simulink model "soccerbot"  (R2017b)
settings: Solver=FixedStepDiscrete  StartTime=0.0  StopTime=10  FixedStep=0.01  RelTol=1e-3
PreLoadFcn:
  | clear;
  | 
  | % Sample times
  | sampleTime = 0.2;
  | 
  | % Control parameters
  | ctrlParam1 = 2;
  | ctrlParam2 = 3.5;
  | 
  | loadIpAddresses;
InitFcn:
  | loadFixedTrajectories;
model workspace (MAT data in the model file):
  SL_ROS_VariableLengthArrays_MaxSizes.CommonInfo.ArrayTruncateAction = 'EmitWarning'
  SL_ROS_VariableLengthArrays_MaxSizes.MsgTypeMap = containers.Map
  SL_ROS_VariableLengthArrays_MaxSizes.MsgTypeMap.serialization.keys = {'sensor_msgs/Image'}
  SL_ROS_VariableLengthArrays_MaxSizes.MsgTypeMap.serialization.values{1}(1).PropertyName = 'Data'
  SL_ROS_VariableLengthArrays_MaxSizes.MsgTypeMap.serialization.values{1}(1).DataType = 'uint8'
  SL_ROS_VariableLengthArrays_MaxSizes.MsgTypeMap.serialization.values{1}(1).MaxLength = 230400
  SL_ROS_VariableLengthArrays_MaxSizes.MsgTypeMap.serialization.values{1}(2).PropertyName = 'Encoding'
  SL_ROS_VariableLengthArrays_MaxSizes.MsgTypeMap.serialization.values{1}(2).DataType = 'uint8'
  SL_ROS_VariableLengthArrays_MaxSizes.MsgTypeMap.serialization.values{1}(2).MaxLength = 128
  SL_ROS_VariableLengthArrays_MaxSizes.MsgTypeMap.serialization.uniformity = 0
  SL_ROS_VariableLengthArrays_MaxSizes.MsgTypeMap.serialization.keyType = 'char'
  SL_ROS_VariableLengthArrays_MaxSizes.MsgTypeMap.serialization.valueType = 'any'
  ctrlParam1 = 1
  ctrlParam2 = 1.5
  sampleTime = 0.01
values from neighbouring files (symbols this model uses):
  findBallTraj = zeros(1000,20)    [loadFixedTrajectories.m]
  getUpBackTraj = getUpBackTraj'    [loadFixedTrajectories.m]
  getUpFrontTraj = getUpFrontTraj'    [loadFixedTrajectories.m]    (also in loadModelData.m)
  motorCalibration = [0;0;0;0;0;0;0;0;0;0;0;0;0;0;0;0;0;0;0;0]    [loadFixedTrajectories.m]    (also in loadRobot.m; soccer_strategy_setup.m)
  prepareToWalkTraj = spline(t, prepareToWalkWayPoints, prepareToWalkTrajTime)'    [loadFixedTrajectories.m]
undefined symbols (not defined in the file or in its folder): customState, DiscIntNeverNeededParam, resting, walkTraj
libraries: simulink x102, robotlib x5, sharedtransform x1, visionsinks x1
(part 1 of 2)
settings Model: Creator=scastro  LastModifiedBy=vuwij
settings OptimizationCC: PassReuseOutputArgsAs=Individual arguments  EfficientMapNaN2IntZero=off  MaxStackSize=64
settings DebuggingCC: ParameterTunabilityLossMsg=error
settings HardwareCC: ProdBitPerPointer=32  ProdBitPerSizeT=32  ProdBitPerPtrDiffT=32  ProdLargestAtomicFloat=None  ProdIntDivRoundTo=Undefined  ProdEndianess=Unspecified  ProdWordSize=32  ProdHWDeviceType=Generic->Unspecified (assume 32-bit Generic)  TargetBitPerLong=64  TargetBitPerPointer=64  TargetBitPerSizeT=64  TargetBitPerPtrDiffT=64  TargetLongLongMode=on  TargetIntDivRoundTo=Zero  TargetEndianess=LittleEndian  TargetWordSize=64  TargetHWDeviceType=MATLAB Host  ProdEqTarget=off
settings SFSimCC: MATLABDynamicMemAlloc=off
settings RTWCC: SystemTargetFile=ert.tlc  HardwareBoard=Robot Operating System (ROS)  TemplateMakefile=ert_default_tmf  GenerateReport=on  Toolchain=Catkin  IncludeHyperlinkInReport=on  LaunchReport=on  TargetLang=C++  GenerateTraceInfo=on  GenerateTraceReport=on  GenerateTraceReportSl=on  GenerateTraceReportSf=on  GenerateTraceReportEml=on
settings CodeAppCC: ForceParamTrailComments=on  IgnoreCustomStorageClasses=off  MaxIdLength=128  OperatorAnnotations=on  SimulinkDataObjDesc=on  SFDataObjDesc=on  InsertBlockDesc=on
settings ERTTargetCC: MultiInstanceERTCode=on  CodeInterfacePackaging=C++ class  RootIOFormat=Structure reference

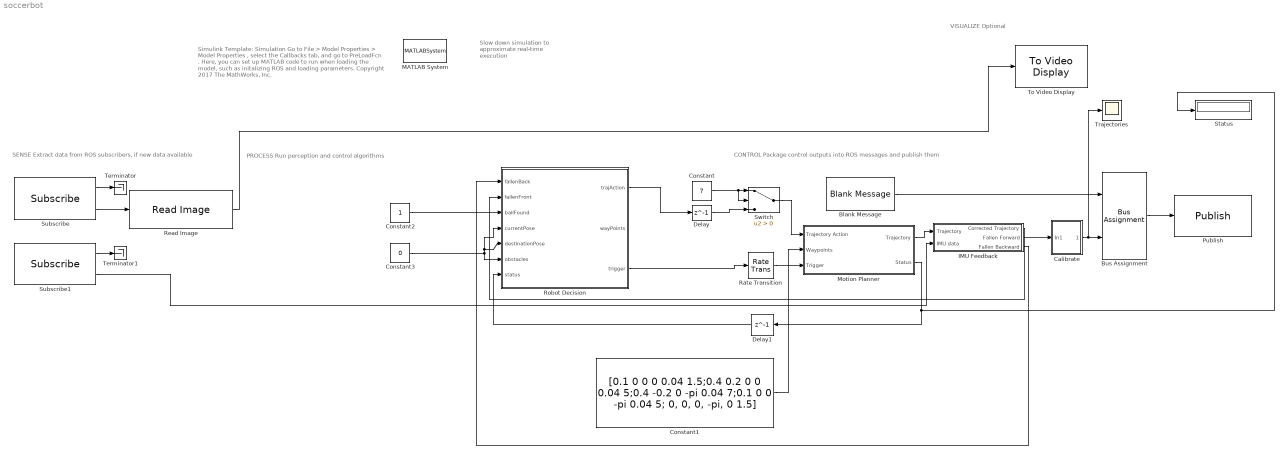
== system soccerbot ==
  note: Simulink Template: Simulation
      |
      | Go to File > Model Properties > Model Properties , select the Callbacks tab, and go to PreLoadFcn .
      |
      | Here, you can set up MATLAB code to run when loading the model, such as initalizing ROS and loading parameters.
      |
      | Copyright 2017 The MathWorks, Inc.
  note: Slow down simulation to approximate real-time execution
  note: PROCESS
      | Run perception and control algorithms
  note: SENSE
      | Extract data from ROS subscribers, if new data available
  note: VISUALIZE
      | Optional
  note: CONTROL
      | Package control outputs into ROS messages and publish them
  Blank Message : robotlib/Blank Message  SourceLibraryInfo=This block requires Robotics System Toolbox  messageType=soccer_msgs/RobotGoal  SampleTime=inf
      settings: SourceProductBaseCode=RO
  Bus Assignment : BusAssignment  AssignedSignals=Trajectories
  Calibrate : Subsystem
  Constant : Constant  Value=7
  Constant1 : Constant  Value=[0.1 0 0 0 0.04 1.5;0.4 0.2 0 0 0.04 5;0.4 -0.2 0 -pi 0.04 7;0.1 0 0 -pi 0.04 5; 0, 0, 0, -pi, 0 1.5]  VectorParams1D=off
  Constant2 : Constant
  Constant3 : Constant  Value=0
  Delay : Delay  DelayLength=1  InitialCondition=1
  Delay1 : Delay  DelayLength=1  InitialCondition=1
  IMU Feedback : Subsystem
  MATLAB System : MATLABSystem  System=ExampleHelperSimulationRateControl  SampleTime=sampleTime
      mask Type: ExampleHelperSimulationRateControl
      mask Display: disp('Rate Control');
  Motion Planner : Subsystem
  Publish : robotlib/Publish  SourceLibraryInfo=This block requires Robotics System Toolbox  topicSource=Select from ROS network  topic=/robotGoal  messageType=soccer_msgs/RobotGoal  messageQueueLength=1
      settings: SourceProductBaseCode=RO
  Rate Transition : RateTransition
  Read Image : robotlib/Read Image  SourceLibraryInfo=This block requires Robotics System Toolbox  MaximumImageSize=[240, 320]  ImageEncoding=rgb8  ShowAlphaOutput=off  ShowErrorCodeOutput=off  VariableSizeOutputs=off
      settings: SourceProductName=Robotics System Toolbox  SourceProductBaseCode=RO
  Robot Decision : Stateflow chart  TreatAsAtomicUnit=on
  Status : Display
  Subscribe : robotlib/Subscribe  SourceLibraryInfo=This block requires Robotics System Toolbox  topicSource=Select from ROS network  topic=/soccerbot/camera1/image_raw  messageType=sensor_msgs/Image  sampleTime=-1  messageQueueLength=1
      settings: SourceProductBaseCode=RO
  Subscribe1 : robotlib/Subscribe  SourceLibraryInfo=This block requires Robotics System Toolbox  topicSource=Select from ROS network  topic=/soccerbot/imu  messageType=sensor_msgs/Imu  sampleTime=-1  messageQueueLength=1
      settings: SourceProductBaseCode=RO
  Switch : Switch  Criteria=u2 > Threshold
  Terminator : Terminator
  Terminator1 : Terminator
  To Video Display : visionsinks/To Video Display  windowSizeMode=Normal  openAtMdlStart=on  fullScreen=off  videoWindowX=838  videoWindowY=73  saveWindowSize=off  videoWindowWidth=487  videoWindowHeight=372  inputColorFormat=RGB  inputType=Obsolete  imagePorts=One multidimensional signal  OutputDevice=On-screen video monitor  dataOrg=Column-major  isWindowOpen=off
      settings: SourceProductName=Computer Vision System Toolbox
  Trajectories : Scope
  wires:
  Subscribe/2 -> Read Image/1
  Subscribe/1 -> Terminator/1
  Calibrate/1(Out1) -> Trajectories/1, Bus Assignment/2
  Bus Assignment/1 -> Publish/1
  Blank Message/1 -> Bus Assignment/1
  Constant1/1 -> Motion Planner/2(Waypoints)
  Constant2/1 -> Robot Decision/3(ballFound)
  Constant3/1 -> Robot Decision/4(currentPose), Robot Decision/5(destinationPose), Robot Decision/6(obstacles)
  Motion Planner/2(Status) -> Status/1, Delay1/1
  Robot Decision/1(trajAction) -> Delay/1
  Rate Transition/1 -> Motion Planner/3(Trigger)
  Robot Decision/3(trigger) -> Rate Transition/1
  Motion Planner/1(Trajectory) -> IMU Feedback/1(Trajectory)
  Read Image/1 -> To Video Display/1
  IMU Feedback/1(Corrected Trajectory) -> Calibrate/1(In1)
  Subscribe1/2 -> IMU Feedback/2(IMU data)
  Subscribe1/1 -> Terminator1/1
  IMU Feedback/2(Fallen Forward) -> Robot Decision/2(fallenFront)
  IMU Feedback/3(Fallen Backward) -> Robot Decision/1(fallenBack)
  Delay/1 -> Switch/3
  Delay1/1 -> Robot Decision/7(status)
  Constant/1 -> Switch/2, Switch/1
  Switch/1 -> Motion Planner/1(Trajectory Action)

== system soccerbot/Calibrate ==
  In1 : Inport
  Add : Sum
  Calibration : Constant  Value=motorCalibration  OutDataTypeStr=single
  Out1 : Outport
  wires:
  In1/1 -> Add/1
  Add/1 -> Out1/1
  Calibration/1 -> Add/2

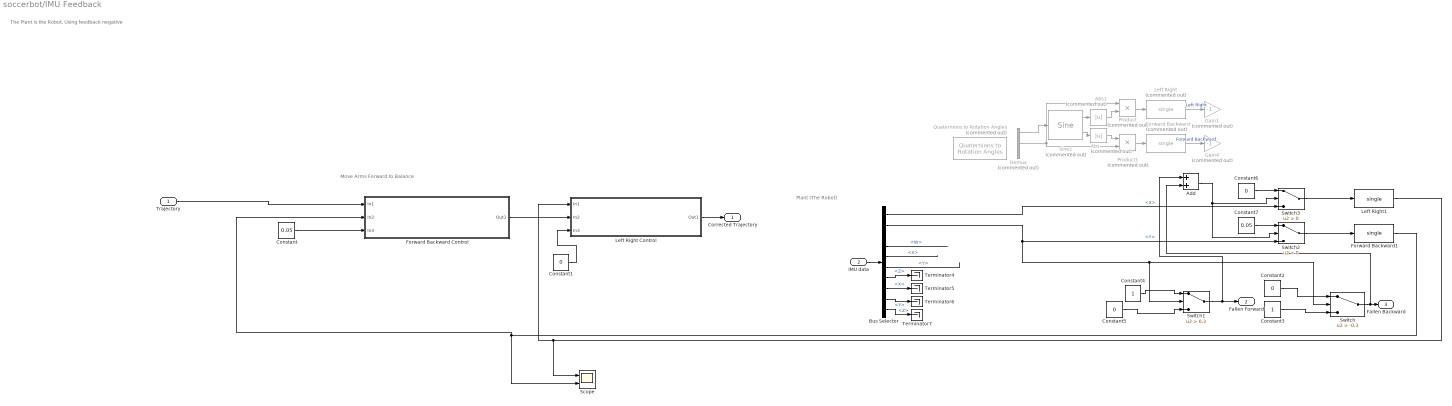
== system soccerbot/IMU Feedback ==
  note: Move Arms Forward to Balance
  note: Plant (The Robot)
  note: The Plant is the Robot, Using feedback negative
  Trajectory : Inport  OutDataTypeStr=single
  IMU data : Inport  Port=2
  Abs : Abs  Commented=on
  Abs1 : Abs  Commented=on
  Add : Sum
  Bus Selector : BusSelector  OutputSignals=Orientation.X,Orientation.Y,Orientation.Z,Orientation.W,AngularVelocity.X,AngularVelocity.Y,AngularVelocity.Z,LinearAcceleration.X,LinearAcceleration.Y,LinearAcceleration.Z
  Constant : Constant  Value=0.05  OutDataTypeStr=single
  Constant1 : Constant  Value=0  OutDataTypeStr=single
  Constant2 : Constant  Value=0
  Constant3 : Constant
  Constant4 : Constant
  Constant5 : Constant  Value=0
  Constant6 : Constant  Value=0
  Constant7 : Constant  Value=0.05
  Demux : Demux  Commented=on  Outputs=3
  Forward Backward : DataTypeConversion  Commented=on  OutDataTypeStr=single
  Forward Backward Control : Subsystem
  Forward Backward1 : DataTypeConversion  OutDataTypeStr=single
  Gain1 : Gain  Commented=on  Gain=-1
  Gain4 : Gain  Commented=on  Gain=-1
  Left Right : DataTypeConversion  Commented=on  OutDataTypeStr=single
  Left Right Control : Subsystem
  Left Right1 : DataTypeConversion  OutDataTypeStr=single
  Product : Product  Commented=on
  Product1 : Product  Commented=on
  Quaternions to Rotation Angles : sharedtransform/Quaternions to Rotation Angles  Commented=on  rotationOrder=ZYZ
      settings: SourceProductBaseCode=AE
  Scope : Scope  NumInputPorts=2
  Sine1 : simulink/Lookup Tables/Sine  Commented=on  Formula=sin(2*pi*u) and cos(2*pi*u)  NumDataPoints=360  OutputWordLength=16  InternalRulePriority=Speed
      settings: SourceProductName=Simulink
  Switch : Switch  Criteria=u2 > Threshold  Threshold=-0.3
  Switch1 : Switch  Criteria=u2 > Threshold  Threshold=0.3
  Switch2 : Switch  Criteria=u2 > Threshold
  Switch3 : Switch  Criteria=u2 > Threshold
  Terminator{4..7} (4 alike) : Terminator
  Corrected Trajectory : Outport
  Fallen Forward : Outport  Port=2
  Fallen Backward : Outport  Port=3
  wires:
  IMU data/1 -> Bus Selector/1
  Bus Selector/5 -> ?  "<X>"
  Bus Selector/6 -> ?  "<Y>"
  Bus Selector/7 -> Terminator4/1  "<Z>"
  Bus Selector/8 -> Terminator5/1  "<X>"
  Bus Selector/9 -> Terminator6/1  "<Y>"
  Bus Selector/10 -> Terminator7/1  "<Z>"
  Trajectory/1 -> Forward Backward Control/1(In1)
  Constant/1 -> Forward Backward Control/3(In3)
  Constant1/1 -> Left Right Control/3(In3)
  Left Right Control/1(Out1) -> Corrected Trajectory/1
  Bus Selector/1 -> Switch3/3  "<X>"
  Bus Selector/2 -> Switch2/3, Switch1/2, Switch/2  "<Y>"
  Bus Selector/4 -> ?  "<W>"
  Switch2/1 -> Forward Backward1/1
  Forward Backward Control/1(Out1) -> Left Right Control/2(In2)
  Switch3/1 -> Left Right1/1
  Demux/1 -> Sine1/1
  Product1/1 -> Forward Backward/1
  Product/1 -> Left Right/1
  Sine1/1 -> Abs1/1
  Forward Backward/1 -> Gain4/1  "Forward Backward"
  Demux/2 -> Product1/2, Product/1
  Abs/1 -> Product1/1
  Left Right/1 -> Gain1/1  "Left RIght"
  Sine1/2 -> Abs/1
  Abs1/1 -> Product/2
  Constant3/1 -> Switch/3
  Constant5/1 -> Switch1/3
  Constant2/1 -> Switch/1
  Constant4/1 -> Switch1/1
  Switch1/1 -> Add/1, Fallen Forward/1
  Constant6/1 -> Switch3/1
  Constant7/1 -> Switch2/1
  Switch/1 -> Add/2, Fallen Backward/1
  Add/1 -> Switch2/2, Switch3/2
  Left Right1/1 -> Left Right Control/1(In1), Scope/1
  Forward Backward1/1 -> Forward Backward Control/2(In2), Scope/2

== system soccerbot/Motion Planner ==
  note: Trajectory Action, 0 for dynamic motion, 1 for fixed motion
  Trajectory Action : Inport
  Waypoints : Inport  Port=2
  Trigger : Inport  Port=3
  Constant : Constant  Value=0  OutDataTypeStr=single
  Constant1 : Constant  Value=0  OutDataTypeStr=single
  Dynamic Trajectories : Subsystem  TreatAsAtomicUnit=on
  Fixed Trajectories : Subsystem  TreatAsAtomicUnit=on
  If : If  IfExpression=u1 == 0
  Merge : Merge
  Merge1 : Merge
  Mux : Mux  Inputs=3
  Trajectory : Outport
  Status : Outport  Port=2
  wires:
  Dynamic Trajectories/1(Out2) -> Merge/1  "Trajectories"
  If/1 -> Dynamic Trajectories/Action
  Trajectory Action/1 -> Fixed Trajectories/1(In1), If/1
  Fixed Trajectories/1(Trajectory) -> Merge/2  "Trajectories"
  If/2 -> Fixed Trajectories/Action
  Waypoints/1 -> Dynamic Trajectories/1(In2)
  Merge/1 -> Mux/1
  Mux/1 -> Trajectory/1
  Constant/1 -> Mux/2
  Constant1/1 -> Mux/3
  Trigger/1 -> Dynamic Trajectories/2(Trigger)
  Merge1/1 -> Status/1
  Fixed Trajectories/2(Status) -> Merge1/2
  Dynamic Trajectories/2(Status) -> Merge1/1

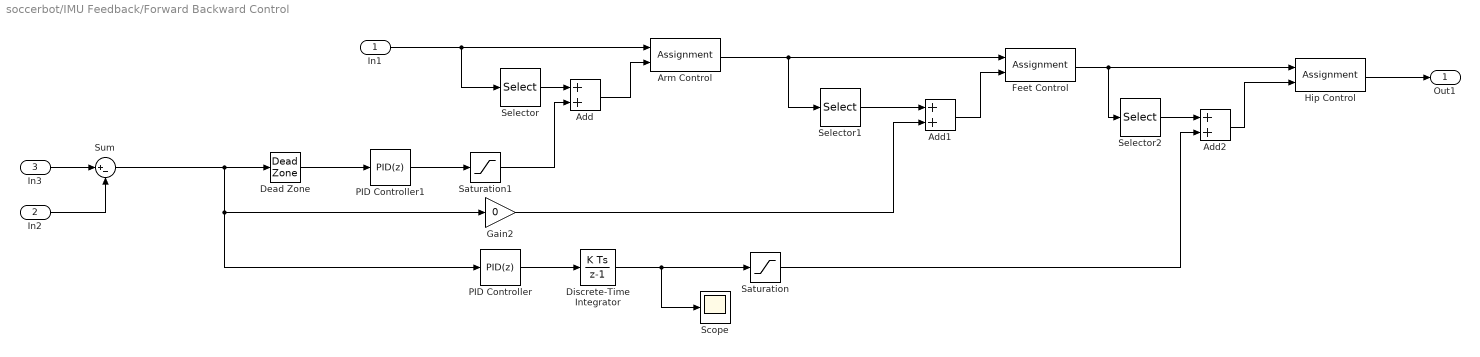
== system soccerbot/IMU Feedback/Forward Backward Control ==
  In1 : Inport
  In2 : Inport  Port=2
  In3 : Inport  Port=3
  Add : Sum
  Add1 : Sum
  Add2 : Sum
  Arm Control : Assignment  DiagnosticForDimensions=Warning  IndexOptions=Index vector (dialog)  Indices=[13 15]  OutputSizes=1
  Dead Zone : DeadZone  LowerValue=-0.03  UpperValue=0.01  SaturateOnIntegerOverflow=on
  Discrete-Time Integrator : DiscreteIntegrator  InitialConditionSetting=State (most efficient)  SampleTime=0.05  ICPrevOutput=DiscIntNeverNeededParam  ICPrevScaledInput=DiscIntNeverNeededParam
  Feet Control : Assignment  DiagnosticForDimensions=Warning  IndexOptions=Index vector (dialog)  Indices=[5 11]  OutputSizes=1
  Gain2 : Gain  Gain=0
  Hip Control : Assignment  DiagnosticForDimensions=Warning  IndexOptions=Index vector (dialog)  Indices=[3 9]  OutputSizes=1
  PID Controller : simulink/Continuous/PID Controller  Controller=PID  TimeDomain=Discrete-time  SampleTime=-1  IntegratorMethod=Forward Euler  FilterMethod=Forward Euler  Form=Parallel  UseFilter=off  ControllerParametersSource=internal  P=1.3  I=0.2  D=0  N=100  InitialConditionSource=internal  InitialConditionForIntegrator=0  InitialConditionForFilter=0  ExternalReset=none  LimitOutput=off  UpperSaturationLimit=inf  LowerSaturationLimit=-inf  LinearizeAsGain=on  AntiWindupMode=none  Kb=1  TrackingMode=off  Kt=1  PParamMin=[]  PParamMax=[]  IParamMin=[]  IParamMax=[]  DParamMin=[]  DParamMax=[]  NParamMin=[]  NParamMax=[]  KbParamMin=[]  KbParamMax=[]  KtParamMin=[]  KtParamMax=[]  POutMin=[]  POutMax=[]  IOutMin=[]  IOutMax=[]  DOutMin=[]  DOutMax=[]  NOutMin=[]  NOutMax=[]  KbOutMin=[]  KbOutMax=[]  KtOutMin=[]  KtOutMax=[]  IntegratorOutMin=[]  IntegratorOutMax=[]  FilterOutMin=[]  FilterOutMax=[]  SumOutMin=[]  SumOutMax=[]  SumI1OutMin=[]  SumI1OutMax=[]  SumI2OutMin=[]  SumI2OutMax=[]  SumI3OutMin=[]  SumI3OutMax=[]  SumDOutMin=[]  SumDOutMax=[]  SaturationOutMin=[]  SaturationOutMax=[]  IntegratorContinuousStateAttributes=''  IntegratorStateMustResolveToSignalObject=off  IntegratorRTWStateStorageClass=Auto  FilterContinuousStateAttributes=''  FilterStateMustResolveToSignalObject=off  FilterRTWStateStorageClass=Auto  DifferentiatorICPrevScaledInput=0  DifferentiatorOutMin=[]  DifferentiatorOutMax=[]  InitialConditionSetting=State (most efficient)  FilterDiffOutCoefMin=[]  FilterDiffOutCoefMax=[]  SumDenOutMin=[]  SumDenOutMax=[]  SumNumOutMin=[]  SumNumOutMax=[]  ReciprocalOutMin=[]  ReciprocalOutMax=[]  DivideOutMin=[]  DivideOutMax=[]  TunerSelectOption=Frequency Response Based
  PID Controller1 : simulink/Continuous/PID Controller  Controller=PID  TimeDomain=Discrete-time  SampleTime=-1  IntegratorMethod=Forward Euler  FilterMethod=Forward Euler  Form=Parallel  UseFilter=off  ControllerParametersSource=internal  P=100  I=1  D=-3  N=100  InitialConditionSource=internal  InitialConditionForIntegrator=0  InitialConditionForFilter=0  ExternalReset=none  LimitOutput=off  UpperSaturationLimit=inf  LowerSaturationLimit=-inf  LinearizeAsGain=on  AntiWindupMode=none  Kb=1  TrackingMode=off  Kt=1  PParamMin=[]  PParamMax=[]  IParamMin=[]  IParamMax=[]  DParamMin=[]  DParamMax=[]  NParamMin=[]  NParamMax=[]  KbParamMin=[]  KbParamMax=[]  KtParamMin=[]  KtParamMax=[]  POutMin=[]  POutMax=[]  IOutMin=[]  IOutMax=[]  DOutMin=[]  DOutMax=[]  NOutMin=[]  NOutMax=[]  KbOutMin=[]  KbOutMax=[]  KtOutMin=[]  KtOutMax=[]  IntegratorOutMin=[]  IntegratorOutMax=[]  FilterOutMin=[]  FilterOutMax=[]  SumOutMin=[]  SumOutMax=[]  SumI1OutMin=[]  SumI1OutMax=[]  SumI2OutMin=[]  SumI2OutMax=[]  SumI3OutMin=[]  SumI3OutMax=[]  SumDOutMin=[]  SumDOutMax=[]  SaturationOutMin=[]  SaturationOutMax=[]  IntegratorContinuousStateAttributes=''  IntegratorStateMustResolveToSignalObject=off  IntegratorRTWStateStorageClass=Auto  FilterContinuousStateAttributes=''  FilterStateMustResolveToSignalObject=off  FilterRTWStateStorageClass=Auto  DifferentiatorICPrevScaledInput=0  DifferentiatorOutMin=[]  DifferentiatorOutMax=[]  InitialConditionSetting=State (most efficient)  FilterDiffOutCoefMin=[]  FilterDiffOutCoefMax=[]  SumDenOutMin=[]  SumDenOutMax=[]  SumNumOutMin=[]  SumNumOutMax=[]  ReciprocalOutMin=[]  ReciprocalOutMax=[]  DivideOutMin=[]  DivideOutMax=[]  TunerSelectOption=Frequency Response Based
  Saturation : Saturate  UpperLimit=1.57  LowerLimit=-0.7
  Saturation1 : Saturate  UpperLimit=1.57
  Scope : Scope
  Selector : Selector  InputPortWidth=20  IndexOptions=Index vector (dialog)  Indices=[13 15]  OutputSizes=1
  Selector1 : Selector  InputPortWidth=20  IndexOptions=Index vector (dialog)  Indices=[5 11]  OutputSizes=1
  Selector2 : Selector  InputPortWidth=20  IndexOptions=Index vector (dialog)  Indices=[3 9]  OutputSizes=1
  Sum : Sum  Inputs=|+-
  Out1 : Outport
  wires:
  In1/1 -> Selector/1, Arm Control/1
  Gain2/1 -> Add1/2
  PID Controller1/1 -> Saturation1/1
  Arm Control/1 -> Feet Control/1, Selector1/1
  Add/1 -> Arm Control/2
  In2/1 -> Sum/2
  Selector/1 -> Add/1
  Add1/1 -> Feet Control/2
  In3/1 -> Sum/1
  Selector1/1 -> Add1/1
  Feet Control/1 -> Selector2/1, Hip Control/1
  Add2/1 -> Hip Control/2
  PID Controller/1 -> Discrete-Time Integrator/1
  Selector2/1 -> Add2/1
  Saturation/1 -> Add2/2
  Hip Control/1 -> Out1/1
  Sum/1 -> Dead Zone/1, Gain2/1, PID Controller/1
  Discrete-Time Integrator/1 -> Scope/1, Saturation/1
  Dead Zone/1 -> PID Controller1/1
  Saturation1/1 -> Add/2

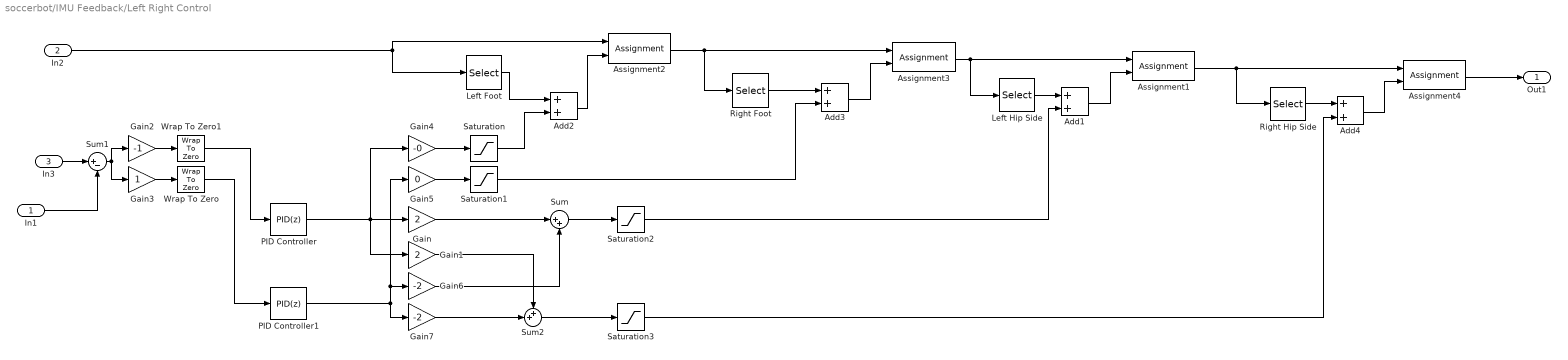
== system soccerbot/IMU Feedback/Left Right Control ==
  In1 : Inport
  In2 : Inport  Port=2
  In3 : Inport  Port=3
  Add{1..4} (4 alike) : Sum
  Assignment1 : Assignment  DiagnosticForDimensions=Warning  IndexOptions=Index vector (dialog)  Indices=2  OutputSizes=1
  Assignment2 : Assignment  DiagnosticForDimensions=Warning  IndexOptions=Index vector (dialog)  Indices=6  OutputSizes=1
  Assignment3 : Assignment  DiagnosticForDimensions=Warning  IndexOptions=Index vector (dialog)  Indices=12  OutputSizes=1
  Assignment4 : Assignment  DiagnosticForDimensions=Warning  IndexOptions=Index vector (dialog)  Indices=8  OutputSizes=1
  Gain : Gain  Gain=2
  Gain1 : Gain  Gain=2
  Gain2 : Gain  Gain=-1
  Gain3 : Gain
  Gain4 : Gain  Gain=-0
  Gain5 : Gain  Gain=0
  Gain6 : Gain  Gain=-2
  Gain7 : Gain  Gain=-2
  Left Foot : Selector  InputPortWidth=20  IndexOptions=Index vector (dialog)  Indices=6  OutputSizes=1
  Left Hip Side : Selector  InputPortWidth=20  IndexOptions=Index vector (dialog)  Indices=2  OutputSizes=1
  PID Controller : simulink/Continuous/PID Controller  Controller=PID  TimeDomain=Discrete-time  SampleTime=-1  IntegratorMethod=Forward Euler  FilterMethod=Forward Euler  Form=Parallel  UseFilter=on  ControllerParametersSource=internal  P=1  I=0  D=0  N=100  InitialConditionSource=internal  InitialConditionForIntegrator=0  InitialConditionForFilter=0  ExternalReset=none  LimitOutput=off  UpperSaturationLimit=inf  LowerSaturationLimit=-inf  LinearizeAsGain=on  AntiWindupMode=none  Kb=1  TrackingMode=off  Kt=1  PParamMin=[]  PParamMax=[]  IParamMin=[]  IParamMax=[]  DParamMin=[]  DParamMax=[]  NParamMin=[]  NParamMax=[]  KbParamMin=[]  KbParamMax=[]  KtParamMin=[]  KtParamMax=[]  POutMin=[]  POutMax=[]  IOutMin=[]  IOutMax=[]  DOutMin=[]  DOutMax=[]  NOutMin=[]  NOutMax=[]  KbOutMin=[]  KbOutMax=[]  KtOutMin=[]  KtOutMax=[]  IntegratorOutMin=[]  IntegratorOutMax=[]  FilterOutMin=[]  FilterOutMax=[]  SumOutMin=[]  SumOutMax=[]  SumI1OutMin=[]  SumI1OutMax=[]  SumI2OutMin=[]  SumI2OutMax=[]  SumI3OutMin=[]  SumI3OutMax=[]  SumDOutMin=[]  SumDOutMax=[]  SaturationOutMin=[]  SaturationOutMax=[]  IntegratorContinuousStateAttributes=''  IntegratorStateMustResolveToSignalObject=off  IntegratorRTWStateStorageClass=Auto  FilterContinuousStateAttributes=''  FilterStateMustResolveToSignalObject=off  FilterRTWStateStorageClass=Auto  DifferentiatorICPrevScaledInput=0  DifferentiatorOutMin=[]  DifferentiatorOutMax=[]  InitialConditionSetting=State (most efficient)  FilterDiffOutCoefMin=[]  FilterDiffOutCoefMax=[]  SumDenOutMin=[]  SumDenOutMax=[]  SumNumOutMin=[]  SumNumOutMax=[]  ReciprocalOutMin=[]  ReciprocalOutMax=[]  DivideOutMin=[]  DivideOutMax=[]  TunerSelectOption=Transfer Function Based (PID Tuner App)
  PID Controller1 : simulink/Continuous/PID Controller  Controller=PID  TimeDomain=Discrete-time  SampleTime=-1  IntegratorMethod=Forward Euler  FilterMethod=Forward Euler  Form=Parallel  UseFilter=on  ControllerParametersSource=internal  P=1  I=0  D=0  N=100  InitialConditionSource=internal  InitialConditionForIntegrator=0  InitialConditionForFilter=0  ExternalReset=none  LimitOutput=off  UpperSaturationLimit=inf  LowerSaturationLimit=-inf  LinearizeAsGain=on  AntiWindupMode=none  Kb=1  TrackingMode=off  Kt=1  PParamMin=[]  PParamMax=[]  IParamMin=[]  IParamMax=[]  DParamMin=[]  DParamMax=[]  NParamMin=[]  NParamMax=[]  KbParamMin=[]  KbParamMax=[]  KtParamMin=[]  KtParamMax=[]  POutMin=[]  POutMax=[]  IOutMin=[]  IOutMax=[]  DOutMin=[]  DOutMax=[]  NOutMin=[]  NOutMax=[]  KbOutMin=[]  KbOutMax=[]  KtOutMin=[]  KtOutMax=[]  IntegratorOutMin=[]  IntegratorOutMax=[]  FilterOutMin=[]  FilterOutMax=[]  SumOutMin=[]  SumOutMax=[]  SumI1OutMin=[]  SumI1OutMax=[]  SumI2OutMin=[]  SumI2OutMax=[]  SumI3OutMin=[]  SumI3OutMax=[]  SumDOutMin=[]  SumDOutMax=[]  SaturationOutMin=[]  SaturationOutMax=[]  IntegratorContinuousStateAttributes=''  IntegratorStateMustResolveToSignalObject=off  IntegratorRTWStateStorageClass=Auto  FilterContinuousStateAttributes=''  FilterStateMustResolveToSignalObject=off  FilterRTWStateStorageClass=Auto  DifferentiatorICPrevScaledInput=0  DifferentiatorOutMin=[]  DifferentiatorOutMax=[]  InitialConditionSetting=State (most efficient)  FilterDiffOutCoefMin=[]  FilterDiffOutCoefMax=[]  SumDenOutMin=[]  SumDenOutMax=[]  SumNumOutMin=[]  SumNumOutMax=[]  ReciprocalOutMin=[]  ReciprocalOutMax=[]  DivideOutMin=[]  DivideOutMax=[]  TunerSelectOption=Transfer Function Based (PID Tuner App)
  Right Foot : Selector  InputPortWidth=20  IndexOptions=Index vector (dialog)  Indices=12  OutputSizes=1
  Right Hip Side : Selector  InputPortWidth=20  IndexOptions=Index vector (dialog)  Indices=8  OutputSizes=1
  Saturation{,1..3} (4 alike) : Saturate  UpperLimit=1  LowerLimit=-1
  Sum : Sum  Inputs=|++
  Sum1 : Sum  Inputs=|+-
  Sum2 : Sum  Inputs=++|
  Wrap To Zero : simulink/Discontinuities/Wrap To Zero  Threshold=0
      settings: SourceProductName=Simulink  SourceProductBaseCode=SL
  Wrap To Zero1 : simulink/Discontinuities/Wrap To Zero  Threshold=0
      settings: SourceProductName=Simulink  SourceProductBaseCode=SL
  Out1 : Outport
  wires:
  In1/1 -> Sum1/2
  In3/1 -> Sum1/1
  Gain3/1 -> Wrap To Zero/1
  Assignment2/1 -> Right Foot/1, Assignment3/1
  Add2/1 -> Assignment2/2
  Gain2/1 -> Wrap To Zero1/1
  Sum1/1 -> Gain2/1, Gain3/1
  Gain5/1 -> Saturation1/1
  Right Foot/1 -> Add3/1
  Left Foot/1 -> Add2/1
  Gain4/1 -> Saturation/1
  Add3/1 -> Assignment3/2
  In2/1 -> Assignment2/1, Left Foot/1
  Wrap To Zero/1 -> PID Controller1/1
  Assignment1/1 -> Right Hip Side/1, Assignment4/1
  Assignment3/1 -> Left Hip Side/1, Assignment1/1
  Assignment4/1 -> Out1/1
  Left Hip Side/1 -> Add1/1
  Add1/1 -> Assignment1/2
  Right Hip Side/1 -> Add4/1
  Add4/1 -> Assignment4/2
  Wrap To Zero1/1 -> PID Controller/1
  Saturation/1 -> Add2/2
  Saturation1/1 -> Add3/2
  Saturation3/1 -> Add4/2
  Saturation2/1 -> Add1/2
  Sum/1 -> Saturation2/1
  Sum2/1 -> Saturation3/1
  Gain/1 -> Sum/1
  Gain1/1 -> Sum2/1
  Gain6/1 -> Sum/2
  Gain7/1 -> Sum2/2
  PID Controller1/1 -> Gain7/1, Gain5/1, Gain6/1
  PID Controller/1 -> Gain4/1, Gain/1, Gain1/1

== system soccerbot/Motion Planner/Dynamic Trajectories ==
  In2 : Inport
  Trigger : Inport  Port=2
  Action Port : ActionPort  ActionType=then
  Constant : Constant  Value=[0,0,0,0,0,0]
  Data Type Conversion : DataTypeConversion  OutDataTypeStr=single
  MATLAB System : MATLABSystem  System=BipedalRobotSystemObject  statusUpdateTimeBeforeEnd=5  SimulateUsing=Interpreted execution
      mask Type: BipedalRobotSystemObject
      mask Display:
      | disp('BipedalRobotSystemObject');
      | port_label('input',1,'waypoints');
      | port_label('input',2,'trigger');
      | port_label('output',1,'trajectories');
      | port_label('output',2,'status');
  Vector Concatenate : Concatenate
  Out2 : Outport
  Status : Outport  Port=2
  wires:
  In2/1 -> MATLAB System/1
  Constant/1 -> Vector Concatenate/2
  Trigger/1 -> MATLAB System/2
  Data Type Conversion/1 -> Out2/1
  Vector Concatenate/1 -> Data Type Conversion/1
  MATLAB System/1 -> Vector Concatenate/1
  MATLAB System/2 -> Status/1

== system soccerbot/Motion Planner/Fixed Trajectories ==
  In1 : Inport
  Action Port : ActionPort  ActionType=else
  "Custom Trajectory " : Subsystem  TreatAsAtomicUnit=on
  Data Type Conversion : DataTypeConversion  OutDataTypeStr=single
  Get Up Back Trajectory : Subsystem  TreatAsAtomicUnit=on
  Get Up Front Trajectory : Subsystem  TreatAsAtomicUnit=on
  If : If  IfExpression=u1 == 0  ElseIfExpressions=u1 == 1, u1 == 2, u1 == 3, u1 == 4, u1 ==5,u1 ==6
  Look For Ball Trajectory : Subsystem  TreatAsAtomicUnit=on
  Merge : Merge  Inputs=8
  Merge1 : Merge  Inputs=8  InitialOutput=0
  Prewalk Trajectory : Subsystem  TreatAsAtomicUnit=on
  Ready Trajectory : Subsystem  TreatAsAtomicUnit=on
  Standing Upright : Subsystem  TreatAsAtomicUnit=on
  Walking Trajectory : Subsystem  TreatAsAtomicUnit=on
  Trajectory : Outport
  Status : Outport  Port=2
  wires:
  Standing Upright/1(Out2) -> Merge/3
  Get Up Back Trajectory/1(Out2) -> Merge/5
  If/4 -> Get Up Front Trajectory/Action
  If/1 -> Walking Trajectory/Action
  Walking Trajectory/1(Trajectory) -> Merge/1
  Data Type Conversion/1 -> Trajectory/1
  Ready Trajectory/1(Out2) -> Merge/2
  Merge/1 -> Data Type Conversion/1
  If/8 -> "Custom Trajectory "/Action
  In1/1 -> If/1
  "Custom Trajectory "/1(Out2) -> Merge/8
  If/5 -> Get Up Back Trajectory/Action
  If/3 -> Standing Upright/Action
  Get Up Front Trajectory/1(Out2) -> Merge/4
  If/2 -> Ready Trajectory/Action
  If/6 -> Look For Ball Trajectory/Action
  Look For Ball Trajectory/1(Out2) -> Merge/6
  If/7 -> Prewalk Trajectory/Action
  Prewalk Trajectory/1(Out2) -> Merge/7
  Prewalk Trajectory/2(Status) -> Merge1/7
  Look For Ball Trajectory/2(Status) -> Merge1/6
  Get Up Back Trajectory/2(Status) -> Merge1/5
  Get Up Front Trajectory/2(Status) -> Merge1/4
  Walking Trajectory/2(Status) -> Merge1/1
  Merge1/1 -> Status/1
  Ready Trajectory/2(Status) -> Merge1/2
  Standing Upright/2(Status) -> Merge1/3
  "Custom Trajectory "/2(Status) -> Merge1/8

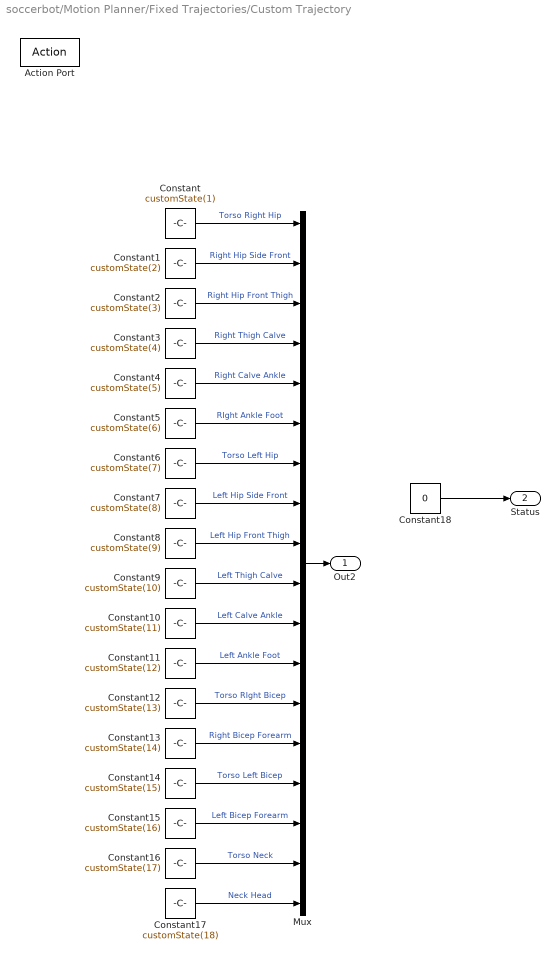
== system soccerbot/Motion Planner/Fixed Trajectories/Custom Trajectory  ==
  Action Port : ActionPort  ActionType=else
  Constant : Constant  Value=customState(1)
  Constant1 : Constant  Value=customState(2)
  Constant10 : Constant  Value=customState(11)
  Constant11 : Constant  Value=customState(12)
  Constant12 : Constant  Value=customState(13)
  Constant13 : Constant  Value=customState(14)
  Constant14 : Constant  Value=customState(15)
  Constant15 : Constant  Value=customState(16)
  Constant16 : Constant  Value=customState(17)
  Constant17 : Constant  Value=customState(18)
  Constant18 : Constant  Value=0
  Constant2 : Constant  Value=customState(3)
  Constant3 : Constant  Value=customState(4)
  Constant4 : Constant  Value=customState(5)
  Constant5 : Constant  Value=customState(6)
  Constant6 : Constant  Value=customState(7)
  Constant7 : Constant  Value=customState(8)
  Constant8 : Constant  Value=customState(9)
  Constant9 : Constant  Value=customState(10)
  Mux : Mux  Inputs=18
  Out2 : Outport
  Status : Outport  Port=2
  wires:
  Constant3/1 -> Mux/4  "Right Thigh Calve"
  Constant12/1 -> Mux/13  "Torso RIght Bicep"
  Constant8/1 -> Mux/9  "Left Hip Front Thigh"
  Constant1/1 -> Mux/2  "Right Hip Side Front"
  Constant14/1 -> Mux/15  "Torso Left Bicep"
  Constant9/1 -> Mux/10  "Left Thigh Calve"
  Constant17/1 -> Mux/18  "Neck Head"
  Constant11/1 -> Mux/12  "Left Ankle Foot"
  Constant16/1 -> Mux/17  "Torso Neck"
  Constant10/1 -> Mux/11  "Left Calve Ankle"
  Constant15/1 -> Mux/16  "Left Bicep Forearm"
  Constant13/1 -> Mux/14  "Right Bicep Forearm"
  Constant/1 -> Mux/1  "Torso Right Hip"
  Mux/1 -> Out2/1
  Constant7/1 -> Mux/8  "Left Hip Side Front"
  Constant2/1 -> Mux/3  "Right Hip Front Thigh"
  Constant6/1 -> Mux/7  "Torso Left Hip"
  Constant4/1 -> Mux/5  "Right Calve Ankle"
  Constant5/1 -> Mux/6  "RIght Ankle Foot"
  Constant18/1 -> Status/1

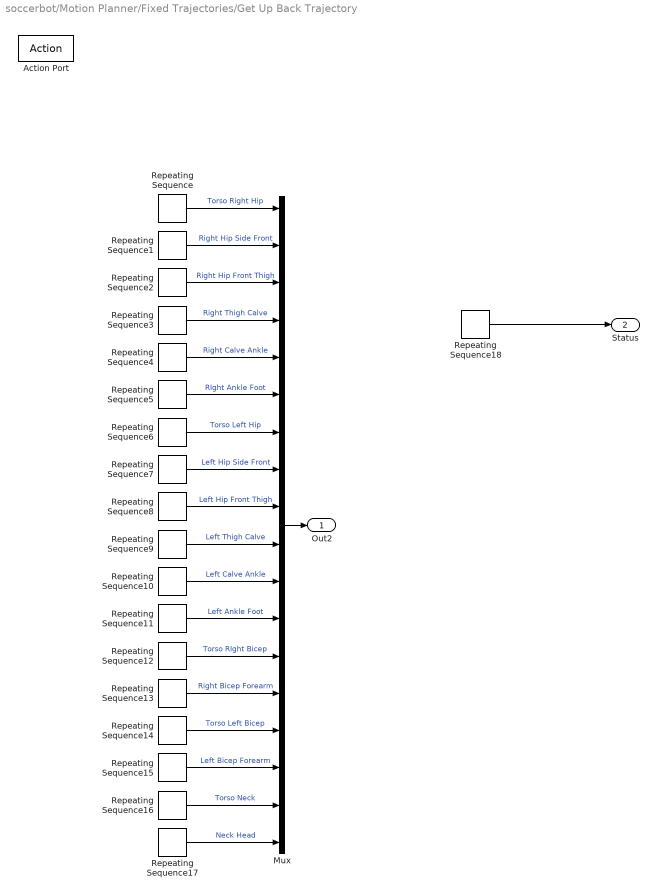
== system soccerbot/Motion Planner/Fixed Trajectories/Get Up Back Trajectory ==
  Action Port : ActionPort  ActionType=elseif
  Mux : Mux  Inputs=18
  Repeating Sequence : simulink/Sources/Repeating Sequence  rep_seq_t=getUpBackTrajTime  rep_seq_y=getUpBackTraj(:,1)
  Repeating Sequence1 : simulink/Sources/Repeating Sequence  rep_seq_t=getUpBackTrajTime  rep_seq_y=getUpBackTraj(:,2)
  Repeating Sequence10 : simulink/Sources/Repeating Sequence  rep_seq_t=getUpBackTrajTime  rep_seq_y=getUpBackTraj(:,11)
  Repeating Sequence11 : simulink/Sources/Repeating Sequence  rep_seq_t=getUpBackTrajTime  rep_seq_y=getUpBackTraj(:,12)
  Repeating Sequence12 : simulink/Sources/Repeating Sequence  rep_seq_t=getUpBackTrajTime  rep_seq_y=getUpBackTraj(:,13)
  Repeating Sequence13 : simulink/Sources/Repeating Sequence  rep_seq_t=getUpBackTrajTime  rep_seq_y=getUpBackTraj(:,14)
  Repeating Sequence14 : simulink/Sources/Repeating Sequence  rep_seq_t=getUpBackTrajTime  rep_seq_y=getUpBackTraj(:,15)
  Repeating Sequence15 : simulink/Sources/Repeating Sequence  rep_seq_t=getUpBackTrajTime  rep_seq_y=getUpBackTraj(:,16)
  Repeating Sequence16 : simulink/Sources/Repeating Sequence  rep_seq_t=getUpBackTrajTime  rep_seq_y=getUpBackTraj(:,17)
  Repeating Sequence17 : simulink/Sources/Repeating Sequence  rep_seq_t=getUpBackTrajTime  rep_seq_y=getUpBackTraj(:,18)
  Repeating Sequence18 : simulink/Sources/Repeating Sequence  rep_seq_t=getUpBackTrajTime  rep_seq_y=getUpBackTrajStatus
  Repeating Sequence2 : simulink/Sources/Repeating Sequence  rep_seq_t=getUpBackTrajTime  rep_seq_y=getUpBackTraj(:,3)
  Repeating Sequence3 : simulink/Sources/Repeating Sequence  rep_seq_t=getUpBackTrajTime  rep_seq_y=getUpBackTraj(:,4)
  Repeating Sequence4 : simulink/Sources/Repeating Sequence  rep_seq_t=getUpBackTrajTime  rep_seq_y=getUpBackTraj(:,5)
  Repeating Sequence5 : simulink/Sources/Repeating Sequence  rep_seq_t=getUpBackTrajTime  rep_seq_y=getUpBackTraj(:,6)
  Repeating Sequence6 : simulink/Sources/Repeating Sequence  rep_seq_t=getUpBackTrajTime  rep_seq_y=getUpBackTraj(:,6)
  Repeating Sequence7 : simulink/Sources/Repeating Sequence  rep_seq_t=getUpBackTrajTime  rep_seq_y=getUpBackTraj(:,8)
  Repeating Sequence8 : simulink/Sources/Repeating Sequence  rep_seq_t=getUpBackTrajTime  rep_seq_y=getUpBackTraj(:,9)
  Repeating Sequence9 : simulink/Sources/Repeating Sequence  rep_seq_t=getUpBackTrajTime  rep_seq_y=getUpBackTraj(:,10)
  Out2 : Outport
  Status : Outport  Port=2
  wires:
  Repeating Sequence3/1 -> Mux/4  "Right Thigh Calve"
  Repeating Sequence12/1 -> Mux/13  "Torso RIght Bicep"
  Repeating Sequence8/1 -> Mux/9  "Left Hip Front Thigh"
  Repeating Sequence1/1 -> Mux/2  "Right Hip Side Front"
  Repeating Sequence14/1 -> Mux/15  "Torso Left Bicep"
  Repeating Sequence9/1 -> Mux/10  "Left Thigh Calve"
  Repeating Sequence17/1 -> Mux/18  "Neck Head"
  Repeating Sequence11/1 -> Mux/12  "Left Ankle Foot"
  Repeating Sequence16/1 -> Mux/17  "Torso Neck"
  Repeating Sequence10/1 -> Mux/11  "Left Calve Ankle"
  Repeating Sequence15/1 -> Mux/16  "Left Bicep Forearm"
  Repeating Sequence13/1 -> Mux/14  "Right Bicep Forearm"
  Repeating Sequence/1 -> Mux/1  "Torso Right Hip"
  Mux/1 -> Out2/1
  Repeating Sequence7/1 -> Mux/8  "Left Hip Side Front"
  Repeating Sequence2/1 -> Mux/3  "Right Hip Front Thigh"
  Repeating Sequence6/1 -> Mux/7  "Torso Left Hip"
  Repeating Sequence4/1 -> Mux/5  "Right Calve Ankle"
  Repeating Sequence5/1 -> Mux/6  "RIght Ankle Foot"
  Repeating Sequence18/1 -> Status/1

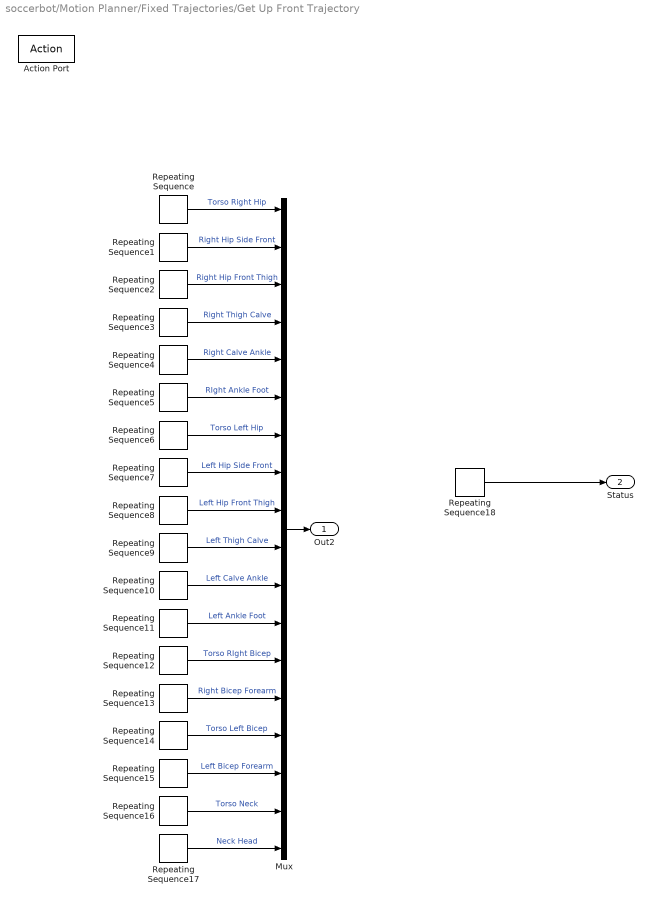
== system soccerbot/Motion Planner/Fixed Trajectories/Get Up Front Trajectory ==
  Action Port : ActionPort  ActionType=elseif
  Mux : Mux  Inputs=18
  Repeating Sequence : simulink/Sources/Repeating Sequence  rep_seq_t=getUpFrontTrajTime  rep_seq_y=getUpFrontTraj(:,1)
  Repeating Sequence1 : simulink/Sources/Repeating Sequence  rep_seq_t=getUpFrontTrajTime  rep_seq_y=getUpFrontTraj(:,2)
  Repeating Sequence10 : simulink/Sources/Repeating Sequence  rep_seq_t=getUpFrontTrajTime  rep_seq_y=getUpFrontTraj(:,11)
  Repeating Sequence11 : simulink/Sources/Repeating Sequence  rep_seq_t=getUpFrontTrajTime  rep_seq_y=getUpFrontTraj(:,12)
  Repeating Sequence12 : simulink/Sources/Repeating Sequence  rep_seq_t=getUpFrontTrajTime  rep_seq_y=getUpFrontTraj(:,13)
  Repeating Sequence13 : simulink/Sources/Repeating Sequence  rep_seq_t=getUpFrontTrajTime  rep_seq_y=getUpFrontTraj(:,14)
  Repeating Sequence14 : simulink/Sources/Repeating Sequence  rep_seq_t=getUpFrontTrajTime  rep_seq_y=getUpFrontTraj(:,15)
  Repeating Sequence15 : simulink/Sources/Repeating Sequence  rep_seq_t=getUpFrontTrajTime  rep_seq_y=getUpFrontTraj(:,16)
  Repeating Sequence16 : simulink/Sources/Repeating Sequence  rep_seq_t=getUpFrontTrajTime  rep_seq_y=getUpFrontTraj(:,17)
  Repeating Sequence17 : simulink/Sources/Repeating Sequence  rep_seq_t=getUpFrontTrajTime  rep_seq_y=getUpFrontTraj(:,18)
  Repeating Sequence18 : simulink/Sources/Repeating Sequence  rep_seq_t=getUpFrontTrajTime  rep_seq_y=getUpFrontTrajStatus
  Repeating Sequence2 : simulink/Sources/Repeating Sequence  rep_seq_t=getUpFrontTrajTime  rep_seq_y=getUpFrontTraj(:,3)
  Repeating Sequence3 : simulink/Sources/Repeating Sequence  rep_seq_t=getUpFrontTrajTime  rep_seq_y=getUpFrontTraj(:,4)
  Repeating Sequence4 : simulink/Sources/Repeating Sequence  rep_seq_t=getUpFrontTrajTime  rep_seq_y=getUpFrontTraj(:,5)
  Repeating Sequence5 : simulink/Sources/Repeating Sequence  rep_seq_t=getUpFrontTrajTime  rep_seq_y=getUpFrontTraj(:,6)
  Repeating Sequence6 : simulink/Sources/Repeating Sequence  rep_seq_t=getUpFrontTrajTime  rep_seq_y=getUpFrontTraj(:,7)
  Repeating Sequence7 : simulink/Sources/Repeating Sequence  rep_seq_t=getUpFrontTrajTime  rep_seq_y=getUpFrontTraj(:,8)
  Repeating Sequence8 : simulink/Sources/Repeating Sequence  rep_seq_t=getUpFrontTrajTime  rep_seq_y=getUpFrontTraj(:,9)
  Repeating Sequence9 : simulink/Sources/Repeating Sequence  rep_seq_t=getUpFrontTrajTime  rep_seq_y=getUpFrontTraj(:,10)
  Out2 : Outport
  Status : Outport  Port=2
  wires:
  Repeating Sequence3/1 -> Mux/4  "Right Thigh Calve"
  Repeating Sequence12/1 -> Mux/13  "Torso RIght Bicep"
  Repeating Sequence8/1 -> Mux/9  "Left Hip Front Thigh"
  Repeating Sequence1/1 -> Mux/2  "Right Hip Side Front"
  Repeating Sequence14/1 -> Mux/15  "Torso Left Bicep"
  Repeating Sequence9/1 -> Mux/10  "Left Thigh Calve"
  Repeating Sequence17/1 -> Mux/18  "Neck Head"
  Repeating Sequence11/1 -> Mux/12  "Left Ankle Foot"
  Repeating Sequence16/1 -> Mux/17  "Torso Neck"
  Repeating Sequence10/1 -> Mux/11  "Left Calve Ankle"
  Repeating Sequence15/1 -> Mux/16  "Left Bicep Forearm"
  Repeating Sequence13/1 -> Mux/14  "Right Bicep Forearm"
  Repeating Sequence/1 -> Mux/1  "Torso Right Hip"
  Mux/1 -> Out2/1
  Repeating Sequence7/1 -> Mux/8  "Left Hip Side Front"
  Repeating Sequence2/1 -> Mux/3  "Right Hip Front Thigh"
  Repeating Sequence6/1 -> Mux/7  "Torso Left Hip"
  Repeating Sequence4/1 -> Mux/5  "Right Calve Ankle"
  Repeating Sequence5/1 -> Mux/6  "RIght Ankle Foot"
  Repeating Sequence18/1 -> Status/1

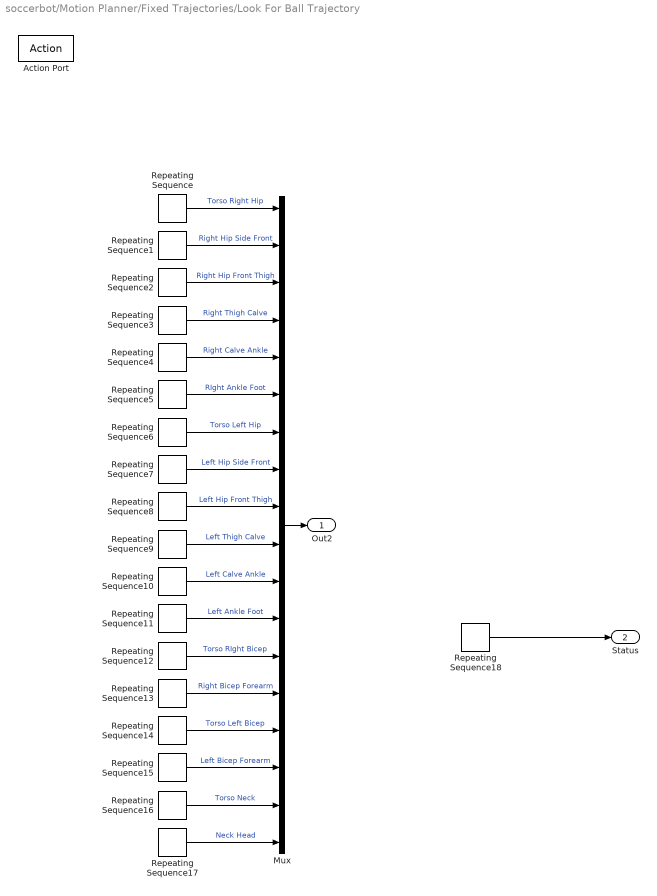
== system soccerbot/Motion Planner/Fixed Trajectories/Look For Ball Trajectory ==
  Action Port : ActionPort  ActionType=elseif
  Mux : Mux  Inputs=18
  Repeating Sequence : simulink/Sources/Repeating Sequence  rep_seq_t=findBallTrajTime  rep_seq_y=findBallTraj(:,1)
  Repeating Sequence1 : simulink/Sources/Repeating Sequence  rep_seq_t=findBallTrajTime  rep_seq_y=findBallTraj(:,2)
  Repeating Sequence10 : simulink/Sources/Repeating Sequence  rep_seq_t=findBallTrajTime  rep_seq_y=findBallTraj(:,11)
  Repeating Sequence11 : simulink/Sources/Repeating Sequence  rep_seq_t=findBallTrajTime  rep_seq_y=findBallTraj(:,12)
  Repeating Sequence12 : simulink/Sources/Repeating Sequence  rep_seq_t=findBallTrajTime  rep_seq_y=findBallTraj(:,13)
  Repeating Sequence13 : simulink/Sources/Repeating Sequence  rep_seq_t=findBallTrajTime  rep_seq_y=findBallTraj(:,14)
  Repeating Sequence14 : simulink/Sources/Repeating Sequence  rep_seq_t=findBallTrajTime  rep_seq_y=findBallTraj(:,15)
  Repeating Sequence15 : simulink/Sources/Repeating Sequence  rep_seq_t=findBallTrajTime  rep_seq_y=findBallTraj(:,16)
  Repeating Sequence16 : simulink/Sources/Repeating Sequence  rep_seq_t=findBallTrajTime  rep_seq_y=findBallTraj(:,17)
  Repeating Sequence17 : simulink/Sources/Repeating Sequence  rep_seq_t=findBallTrajTime  rep_seq_y=findBallTraj(:,18)
  Repeating Sequence18 : simulink/Sources/Repeating Sequence  rep_seq_t=findBallTrajTime  rep_seq_y=findBallTrajStatus
  Repeating Sequence2 : simulink/Sources/Repeating Sequence  rep_seq_t=findBallTrajTime  rep_seq_y=findBallTraj(:,3)
  Repeating Sequence3 : simulink/Sources/Repeating Sequence  rep_seq_t=findBallTrajTime  rep_seq_y=findBallTraj(:,4)
  Repeating Sequence4 : simulink/Sources/Repeating Sequence  rep_seq_t=findBallTrajTime  rep_seq_y=findBallTraj(:,5)
  Repeating Sequence5 : simulink/Sources/Repeating Sequence  rep_seq_t=findBallTrajTime  rep_seq_y=findBallTraj(:,6)
  Repeating Sequence6 : simulink/Sources/Repeating Sequence  rep_seq_t=findBallTrajTime  rep_seq_y=findBallTraj(:,7)
  Repeating Sequence7 : simulink/Sources/Repeating Sequence  rep_seq_t=findBallTrajTime  rep_seq_y=findBallTraj(:,8)
  Repeating Sequence8 : simulink/Sources/Repeating Sequence  rep_seq_t=findBallTrajTime  rep_seq_y=findBallTraj(:,9)
  Repeating Sequence9 : simulink/Sources/Repeating Sequence  rep_seq_t=findBallTrajTime  rep_seq_y=findBallTraj(:,10)
  Out2 : Outport
  Status : Outport  Port=2
  wires:
  Repeating Sequence3/1 -> Mux/4  "Right Thigh Calve"
  Repeating Sequence12/1 -> Mux/13  "Torso RIght Bicep"
  Repeating Sequence8/1 -> Mux/9  "Left Hip Front Thigh"
  Repeating Sequence1/1 -> Mux/2  "Right Hip Side Front"
  Repeating Sequence14/1 -> Mux/15  "Torso Left Bicep"
  Repeating Sequence9/1 -> Mux/10  "Left Thigh Calve"
  Repeating Sequence17/1 -> Mux/18  "Neck Head"
  Repeating Sequence11/1 -> Mux/12  "Left Ankle Foot"
  Repeating Sequence16/1 -> Mux/17  "Torso Neck"
  Repeating Sequence10/1 -> Mux/11  "Left Calve Ankle"
  Repeating Sequence15/1 -> Mux/16  "Left Bicep Forearm"
  Repeating Sequence13/1 -> Mux/14  "Right Bicep Forearm"
  Repeating Sequence/1 -> Mux/1  "Torso Right Hip"
  Mux/1 -> Out2/1
  Repeating Sequence7/1 -> Mux/8  "Left Hip Side Front"
  Repeating Sequence2/1 -> Mux/3  "Right Hip Front Thigh"
  Repeating Sequence6/1 -> Mux/7  "Torso Left Hip"
  Repeating Sequence4/1 -> Mux/5  "Right Calve Ankle"
  Repeating Sequence5/1 -> Mux/6  "RIght Ankle Foot"
  Repeating Sequence18/1 -> Status/1

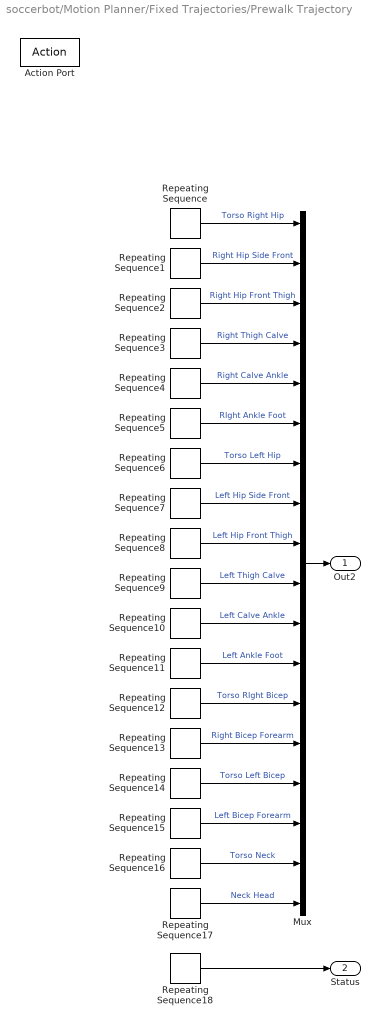
== system soccerbot/Motion Planner/Fixed Trajectories/Prewalk Trajectory ==
  Action Port : ActionPort  ActionType=elseif
  Mux : Mux  Inputs=18
  Repeating Sequence : simulink/Sources/Repeating Sequence  rep_seq_t=prepareToWalkTrajTime  rep_seq_y=prepareToWalkTraj(:,1)
  Repeating Sequence1 : simulink/Sources/Repeating Sequence  rep_seq_t=prepareToWalkTrajTime  rep_seq_y=prepareToWalkTraj(:,2)
  Repeating Sequence10 : simulink/Sources/Repeating Sequence  rep_seq_t=prepareToWalkTrajTime  rep_seq_y=prepareToWalkTraj(:,11)
  Repeating Sequence11 : simulink/Sources/Repeating Sequence  rep_seq_t=prepareToWalkTrajTime  rep_seq_y=prepareToWalkTraj(:,12)
  Repeating Sequence12 : simulink/Sources/Repeating Sequence  rep_seq_t=prepareToWalkTrajTime  rep_seq_y=prepareToWalkTraj(:,13)
  Repeating Sequence13 : simulink/Sources/Repeating Sequence  rep_seq_t=prepareToWalkTrajTime  rep_seq_y=prepareToWalkTraj(:,14)
  Repeating Sequence14 : simulink/Sources/Repeating Sequence  rep_seq_t=prepareToWalkTrajTime  rep_seq_y=prepareToWalkTraj(:,15)
  Repeating Sequence15 : simulink/Sources/Repeating Sequence  rep_seq_t=prepareToWalkTrajTime  rep_seq_y=prepareToWalkTraj(:,16)
  Repeating Sequence16 : simulink/Sources/Repeating Sequence  rep_seq_t=prepareToWalkTrajTime  rep_seq_y=prepareToWalkTraj(:,17)
  Repeating Sequence17 : simulink/Sources/Repeating Sequence  rep_seq_t=prepareToWalkTrajTime  rep_seq_y=prepareToWalkTraj(:,18)
  Repeating Sequence18 : simulink/Sources/Repeating Sequence  rep_seq_t=prepareToWalkTrajTime  rep_seq_y=prepareToWalkTrajStatus
  Repeating Sequence2 : simulink/Sources/Repeating Sequence  rep_seq_t=prepareToWalkTrajTime  rep_seq_y=prepareToWalkTraj(:,3)
  Repeating Sequence3 : simulink/Sources/Repeating Sequence  rep_seq_t=prepareToWalkTrajTime  rep_seq_y=prepareToWalkTraj(:,4)
  Repeating Sequence4 : simulink/Sources/Repeating Sequence  rep_seq_t=prepareToWalkTrajTime  rep_seq_y=prepareToWalkTraj(:,5)
  Repeating Sequence5 : simulink/Sources/Repeating Sequence  rep_seq_t=prepareToWalkTrajTime  rep_seq_y=prepareToWalkTraj(:,6)
  Repeating Sequence6 : simulink/Sources/Repeating Sequence  rep_seq_t=prepareToWalkTrajTime  rep_seq_y=prepareToWalkTraj(:,7)
  Repeating Sequence7 : simulink/Sources/Repeating Sequence  rep_seq_t=prepareToWalkTrajTime  rep_seq_y=prepareToWalkTraj(:,8)
  Repeating Sequence8 : simulink/Sources/Repeating Sequence  rep_seq_t=prepareToWalkTrajTime  rep_seq_y=prepareToWalkTraj(:,9)
  Repeating Sequence9 : simulink/Sources/Repeating Sequence  rep_seq_t=prepareToWalkTrajTime  rep_seq_y=prepareToWalkTraj(:,10)
  Out2 : Outport
  Status : Outport  Port=2
  wires:
  Repeating Sequence3/1 -> Mux/4  "Right Thigh Calve"
  Repeating Sequence12/1 -> Mux/13  "Torso RIght Bicep"
  Repeating Sequence8/1 -> Mux/9  "Left Hip Front Thigh"
  Repeating Sequence1/1 -> Mux/2  "Right Hip Side Front"
  Repeating Sequence14/1 -> Mux/15  "Torso Left Bicep"
  Repeating Sequence9/1 -> Mux/10  "Left Thigh Calve"
  Repeating Sequence17/1 -> Mux/18  "Neck Head"
  Repeating Sequence11/1 -> Mux/12  "Left Ankle Foot"
  Repeating Sequence16/1 -> Mux/17  "Torso Neck"
  Repeating Sequence10/1 -> Mux/11  "Left Calve Ankle"
  Repeating Sequence15/1 -> Mux/16  "Left Bicep Forearm"
  Repeating Sequence13/1 -> Mux/14  "Right Bicep Forearm"
  Repeating Sequence/1 -> Mux/1  "Torso Right Hip"
  Mux/1 -> Out2/1
  Repeating Sequence7/1 -> Mux/8  "Left Hip Side Front"
  Repeating Sequence2/1 -> Mux/3  "Right Hip Front Thigh"
  Repeating Sequence6/1 -> Mux/7  "Torso Left Hip"
  Repeating Sequence4/1 -> Mux/5  "Right Calve Ankle"
  Repeating Sequence5/1 -> Mux/6  "RIght Ankle Foot"
  Repeating Sequence18/1 -> Status/1

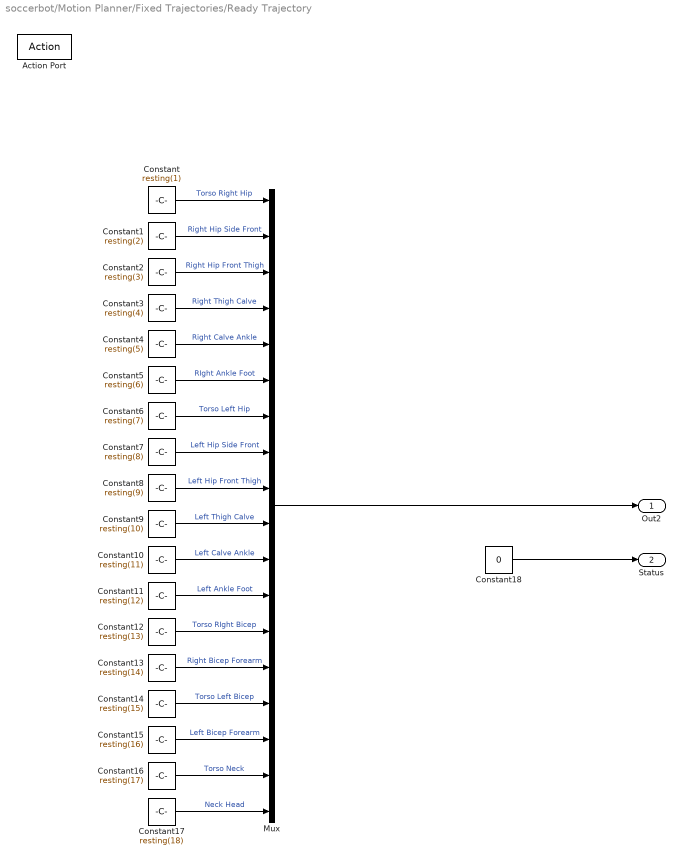
== system soccerbot/Motion Planner/Fixed Trajectories/Ready Trajectory ==
  Action Port : ActionPort  ActionType=elseif
  Constant : Constant  Value=resting(1)
  Constant1 : Constant  Value=resting(2)
  Constant10 : Constant  Value=resting(11)
  Constant11 : Constant  Value=resting(12)
  Constant12 : Constant  Value=resting(13)
  Constant13 : Constant  Value=resting(14)
  Constant14 : Constant  Value=resting(15)
  Constant15 : Constant  Value=resting(16)
  Constant16 : Constant  Value=resting(17)
  Constant17 : Constant  Value=resting(18)
  Constant18 : Constant  Value=0
  Constant2 : Constant  Value=resting(3)
  Constant3 : Constant  Value=resting(4)
  Constant4 : Constant  Value=resting(5)
  Constant5 : Constant  Value=resting(6)
  Constant6 : Constant  Value=resting(7)
  Constant7 : Constant  Value=resting(8)
  Constant8 : Constant  Value=resting(9)
  Constant9 : Constant  Value=resting(10)
  Mux : Mux  Inputs=18
  Out2 : Outport
  Status : Outport  Port=2
  wires:
  Constant3/1 -> Mux/4  "Right Thigh Calve"
  Constant12/1 -> Mux/13  "Torso RIght Bicep"
  Constant8/1 -> Mux/9  "Left Hip Front Thigh"
  Constant1/1 -> Mux/2  "Right Hip Side Front"
  Constant14/1 -> Mux/15  "Torso Left Bicep"
  Constant9/1 -> Mux/10  "Left Thigh Calve"
  Constant17/1 -> Mux/18  "Neck Head"
  Constant11/1 -> Mux/12  "Left Ankle Foot"
  Constant16/1 -> Mux/17  "Torso Neck"
  Constant10/1 -> Mux/11  "Left Calve Ankle"
  Constant15/1 -> Mux/16  "Left Bicep Forearm"
  Constant13/1 -> Mux/14  "Right Bicep Forearm"
  Constant/1 -> Mux/1  "Torso Right Hip"
  Constant7/1 -> Mux/8  "Left Hip Side Front"
  Constant2/1 -> Mux/3  "Right Hip Front Thigh"
  Constant6/1 -> Mux/7  "Torso Left Hip"
  Constant4/1 -> Mux/5  "Right Calve Ankle"
  Constant5/1 -> Mux/6  "RIght Ankle Foot"
  Mux/1 -> Out2/1
  Constant18/1 -> Status/1

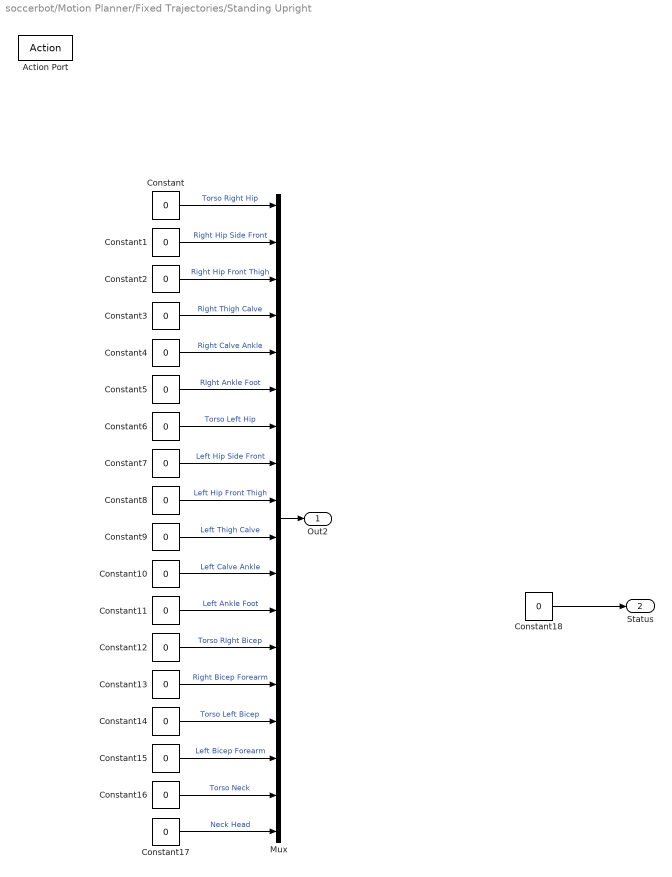
== system soccerbot/Motion Planner/Fixed Trajectories/Standing Upright ==
  Action Port : ActionPort  ActionType=elseif
  Constant{,1..18} (19 alike) : Constant  Value=0
  Mux : Mux  Inputs=18
  Out2 : Outport
  Status : Outport  Port=2
  wires:
  Constant3/1 -> Mux/4  "Right Thigh Calve"
  Constant12/1 -> Mux/13  "Torso RIght Bicep"
  Constant8/1 -> Mux/9  "Left Hip Front Thigh"
  Constant1/1 -> Mux/2  "Right Hip Side Front"
  Constant14/1 -> Mux/15  "Torso Left Bicep"
  Constant9/1 -> Mux/10  "Left Thigh Calve"
  Constant17/1 -> Mux/18  "Neck Head"
  Constant11/1 -> Mux/12  "Left Ankle Foot"
  Constant16/1 -> Mux/17  "Torso Neck"
  Constant10/1 -> Mux/11  "Left Calve Ankle"
  Constant15/1 -> Mux/16  "Left Bicep Forearm"
  Constant13/1 -> Mux/14  "Right Bicep Forearm"
  Constant/1 -> Mux/1  "Torso Right Hip"
  Mux/1 -> Out2/1
  Constant7/1 -> Mux/8  "Left Hip Side Front"
  Constant2/1 -> Mux/3  "Right Hip Front Thigh"
  Constant6/1 -> Mux/7  "Torso Left Hip"
  Constant4/1 -> Mux/5  "Right Calve Ankle"
  Constant5/1 -> Mux/6  "RIght Ankle Foot"
  Constant18/1 -> Status/1

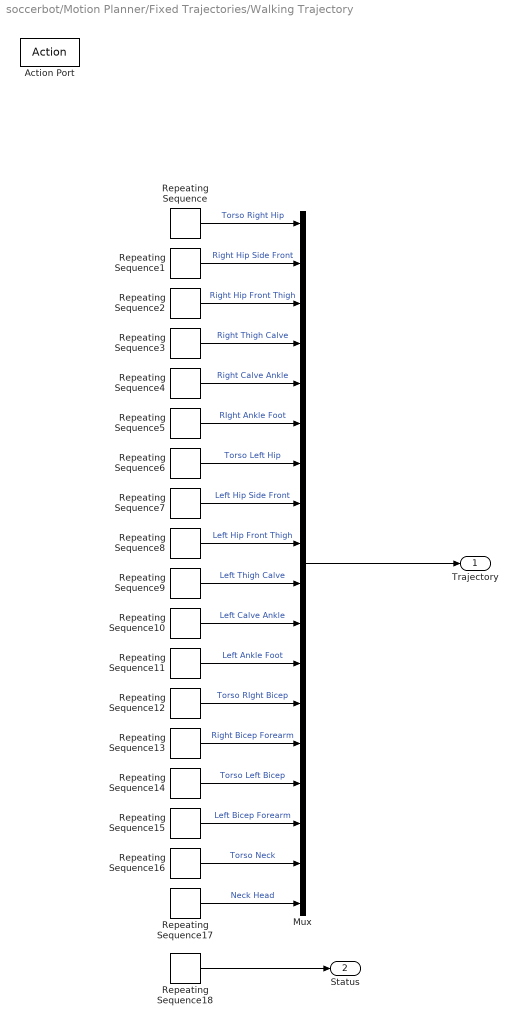
== system soccerbot/Motion Planner/Fixed Trajectories/Walking Trajectory ==
  Action Port : ActionPort  ActionType=then
  Mux : Mux  Inputs=18
  Repeating Sequence : simulink/Sources/Repeating Sequence  rep_seq_t=walkTrajTime  rep_seq_y=walkTraj(:,1)
  Repeating Sequence1 : simulink/Sources/Repeating Sequence  rep_seq_t=walkTrajTime  rep_seq_y=walkTraj(:,2)
  Repeating Sequence10 : simulink/Sources/Repeating Sequence  rep_seq_t=walkTrajTime  rep_seq_y=walkTraj(:,11)
  Repeating Sequence11 : simulink/Sources/Repeating Sequence  rep_seq_t=walkTrajTime  rep_seq_y=walkTraj(:,12)
  Repeating Sequence12 : simulink/Sources/Repeating Sequence  rep_seq_t=walkTrajTime  rep_seq_y=walkTraj(:,13)
  Repeating Sequence13 : simulink/Sources/Repeating Sequence  rep_seq_t=walkTrajTime  rep_seq_y=walkTraj(:,14)
  Repeating Sequence14 : simulink/Sources/Repeating Sequence  rep_seq_t=walkTrajTime  rep_seq_y=walkTraj(:,15)
  Repeating Sequence15 : simulink/Sources/Repeating Sequence  rep_seq_t=walkTrajTime  rep_seq_y=walkTraj(:,16)
  Repeating Sequence16 : simulink/Sources/Repeating Sequence  rep_seq_t=walkTrajTime  rep_seq_y=walkTraj(:,17)
  Repeating Sequence17 : simulink/Sources/Repeating Sequence  rep_seq_t=walkTrajTime  rep_seq_y=walkTraj(:,18)
  Repeating Sequence18 : simulink/Sources/Repeating Sequence  rep_seq_t=walkTrajTime  rep_seq_y=walkTrajStatus
  Repeating Sequence2 : simulink/Sources/Repeating Sequence  rep_seq_t=walkTrajTime  rep_seq_y=walkTraj(:,3)
  Repeating Sequence3 : simulink/Sources/Repeating Sequence  rep_seq_t=walkTrajTime  rep_seq_y=walkTraj(:,4)
  Repeating Sequence4 : simulink/Sources/Repeating Sequence  rep_seq_t=walkTrajTime  rep_seq_y=walkTraj(:,5)
  Repeating Sequence5 : simulink/Sources/Repeating Sequence  rep_seq_t=walkTrajTime  rep_seq_y=walkTraj(:,6)
  Repeating Sequence6 : simulink/Sources/Repeating Sequence  rep_seq_t=walkTrajTime  rep_seq_y=walkTraj(:,7)
  Repeating Sequence7 : simulink/Sources/Repeating Sequence  rep_seq_t=walkTrajTime  rep_seq_y=walkTraj(:,8)
  Repeating Sequence8 : simulink/Sources/Repeating Sequence  rep_seq_t=walkTrajTime  rep_seq_y=walkTraj(:,9)
  Repeating Sequence9 : simulink/Sources/Repeating Sequence  rep_seq_t=walkTrajTime  rep_seq_y=walkTraj(:,10)
  Trajectory : Outport
  Status : Outport  Port=2
  wires:
  Repeating Sequence3/1 -> Mux/4  "Right Thigh Calve"
  Repeating Sequence12/1 -> Mux/13  "Torso RIght Bicep"
  Repeating Sequence8/1 -> Mux/9  "Left Hip Front Thigh"
  Repeating Sequence1/1 -> Mux/2  "Right Hip Side Front"
  Repeating Sequence14/1 -> Mux/15  "Torso Left Bicep"
  Repeating Sequence9/1 -> Mux/10  "Left Thigh Calve"
  Repeating Sequence17/1 -> Mux/18  "Neck Head"
  Repeating Sequence11/1 -> Mux/12  "Left Ankle Foot"
  Repeating Sequence16/1 -> Mux/17  "Torso Neck"
  Repeating Sequence10/1 -> Mux/11  "Left Calve Ankle"
  Repeating Sequence15/1 -> Mux/16  "Left Bicep Forearm"
  Repeating Sequence13/1 -> Mux/14  "Right Bicep Forearm"
  Repeating Sequence/1 -> Mux/1  "Torso Right Hip"
  Mux/1 -> Trajectory/1
  Repeating Sequence7/1 -> Mux/8  "Left Hip Side Front"
  Repeating Sequence2/1 -> Mux/3  "Right Hip Front Thigh"
  Repeating Sequence6/1 -> Mux/7  "Torso Left Hip"
  Repeating Sequence4/1 -> Mux/5  "Right Calve Ankle"
  Repeating Sequence5/1 -> Mux/6  "RIght Ankle Foot"
  Repeating Sequence18/1 -> Status/1
